simulink model "MDL_Tstribeck"  (R2023a)
settings: Solver=ode4  StartTime=0.0  StopTime=end_time  FixedStep=dt  MaxStep=0.001  RelTol=1e-3
values from neighbouring files (symbols this model uses):
  dt = 0.001    [anim_sim_script.m]
  IC = [x_ic, theta_ic, D_x_ic, D_theta_ic]'    [anim_sim_script.m]
settings Model: Creator=Adam  LastModifiedBy=Adam
settings SolverCC: AlgebraicLoopSolver=TrustRegion
settings DataIOCC: SaveOutput=off  SignalLogging=off  DSMLogging=off
settings DebuggingCC: AlgebraicLoopMsg=none  UnconnectedInputMsg=warning  UnconnectedOutputMsg=warning  UnconnectedLineMsg=warning
settings ModelReferenceCC: EnableRefExpFcnMdlSchedulingChecks=on
settings RTWCC: DLArmComputeVersion=19.05

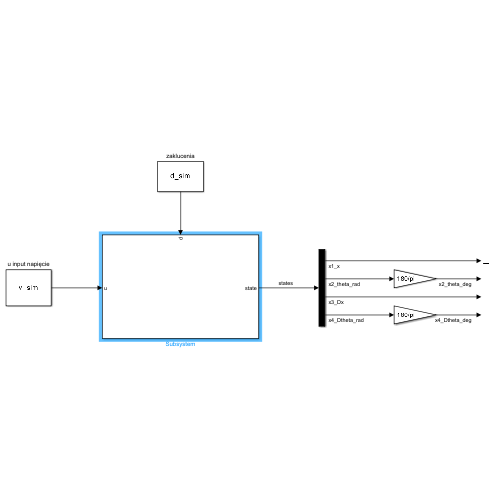
[thumbnail: Simulink's stored preview of the top-level diagram]
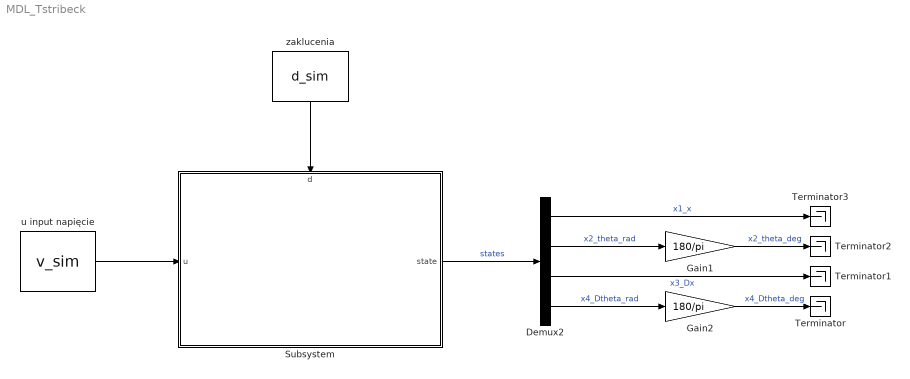
== system MDL_Tstribeck ==
  Demux2 : Demux
  Gain1 : Gain  Gain=180/pi
  Gain2 : Gain  Gain=180/pi
  Subsystem : Subsystem
      settings: PortSchema="{\"entries\":[{\"content\":{\"sides\":[{\"content\":{\"connectorIds\":[\"In1\"]},\"type\":\"ConnectorPlacement.EquallySpacedRectSide\",\"uuid\":\"016ea867-ddd8-4e4e-bab4-0d2197a0eca8\"},{\"content\":{\"connectorIds\":[\"Out1\"],\"side\":\"RIGHT\"},\"type\":\"ConnectorPlacement.EquallySpacedRectSide\",\"uuid\":\"d1d8bb54-69f3-4222-bf08-1602f551b392\"},{\"content\":{\"connectorIds\":[\"In2\"],\"side\":\"TOP\"},\"type\":\"ConnectorPlacement.EquallySpacedRectSide\",\"uuid\":\"6a1bb223-f200-4a07-967e-0b0401ecc4d0\"}]},\"type\":\"ConnectorPlacement.EquallySpacedConnector\",\"uuid\":\"1caa5d0d-86db-4cb9-b67b-4da6d1c4b76b\"}],\"packageUris\":[\"http://schema.mathworks.com/mf0/Connector/R2020b\"],\"version\":\"1.0\"}"
  Terminator{,1..3} (4 alike) : Terminator
  u input napięcie : FromWorkspace  VariableName=v_sim  SampleTime=dt
  zaklucenia : FromWorkspace  VariableName=d_sim  SampleTime=dt
  wires:
  Gain2/1 -> Terminator/1  "x4_Dtheta_deg"
  Demux2/4 -> Gain2/1  "x4_Dtheta_rad"
  Demux2/3 -> Terminator1/1  "x3_Dx"
  Demux2/2 -> Gain1/1  "x2_theta_rad"
  Demux2/1 -> Terminator3/1  "x1_x"
  Gain1/1 -> Terminator2/1  "x2_theta_deg"
  Subsystem/1(state) -> Demux2/1  "states"
  u input napięcie/1 -> Subsystem/1(u)
  zaklucenia/1 -> Subsystem/2(d)

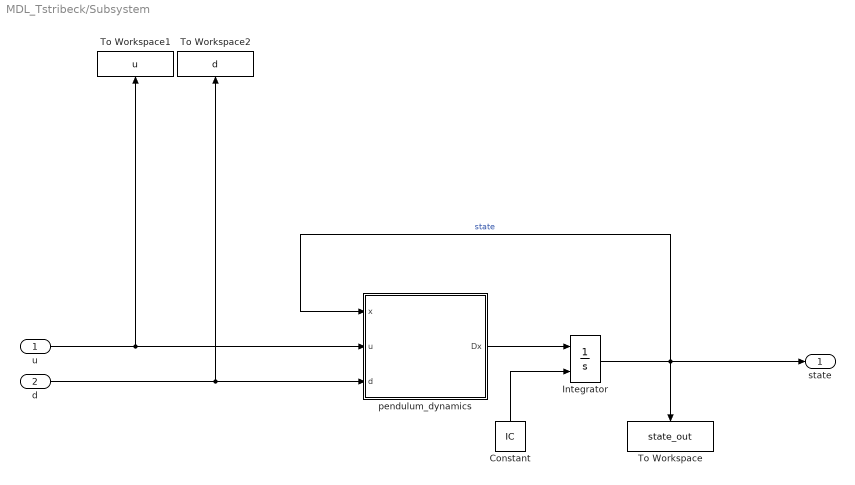
== system MDL_Tstribeck/Subsystem ==
  u : Inport
  d : Inport  Port=2
  Constant : Constant  Value=IC
  Integrator : Integrator  InitialConditionSource=external
  To Workspace : ToWorkspace  VariableName=state_out  SampleTime=-1
      settings: Save2DSignal=2-D array (concatenate along first dimension)
  To Workspace1 : ToWorkspace  VariableName=u  SampleTime=-1
  To Workspace2 : ToWorkspace  VariableName=d  SampleTime=-1
  pendulum_dynamics : MATLAB Function  TreatAsAtomicUnit=on
  state : Outport
  wires:
  Integrator/1 -> pendulum_dynamics/1(x), state/1, To Workspace/1  "state"
  u/1 -> pendulum_dynamics/2(u), To Workspace1/1
  pendulum_dynamics/1(Dx) -> Integrator/1
  Constant/1 -> Integrator/2
  d/1 -> pendulum_dynamics/3(d), To Workspace2/1

== matlab function MDL_Tstribeck/Subsystem/pendulum_dynamics ==
  data: x input; u input; d input; Dx output; params_stribeck parameter
function Dx = dynamika_wahadla(x, u, d, params_stribeck)
% x : stan
% u : input - napięcie
%
% params scope: "parameters"
%

% State, function input: x = [x Dx theta Dtheta]'
x1 = x(1);
x2 = x(2);
x3 = x(3);
x4 = x(4);

params_stribeck = num2cell(params_stribeck);
[M, mc, mp, Lp, Lc, g, b_stribeck, gamma, mr, Mt, L, Jcm, Jt, alpha, beta, miu_c, miu_s, vs, i_, delta] = params_stribeck{:};

% Equations for pendulum dynamics
Ff = (miu_c + (miu_s-miu_c)*exp(-(x3/vs)^i_)) * Mt*g*tanh(delta*x3) + b_stribeck*x3;
Fi = alpha*u - beta*x3;
A = d*cos(x2) - Ff + L*mr*x4^2*sin(x2) + Fi;
B = d*Lc + L*g*mr*sin(x2) - gamma*x4;
DEN = Jt*Mt - (L*mr*cos(x2))^2;

ddt_x1 = x3;
ddt_x2 = x4;
ddt_x3 = (Jt*A - L*mr*cos(x2)*B) / DEN;
ddt_x4 = (Mt*B - L*mr*cos(x2)*A) / DEN;

% output
Dx = [ddt_x1 ddt_x2 ddt_x3 ddt_x4]';

end
